simulink model "equation_circle"  (R2021a)
settings: Solver=VariableStepAuto  StartTime=0.0  StopTime=10.0  RelTol=1e-3
libraries: simulink x3
settings Model: Creator=Aula  LastModifiedBy=Aula

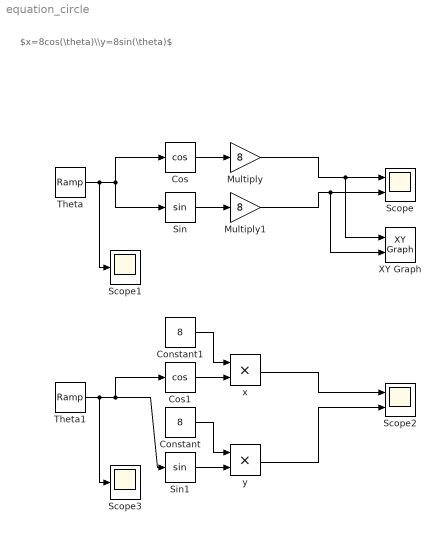
== system equation_circle ==
  note: $x=8cos(\theta)\\y=8sin(\theta)$
  Constant : Constant  Value=8
  Constant1 : Constant  Value=8
  Cos : Trigonometry  Operator=cos
  Cos1 : Trigonometry  Operator=cos
  Multiply : Gain  Gain=8
  Multiply1 : Gain  Gain=8
  Scope : Scope  NumInputPorts=2
  Scope1 : Scope
  Scope2 : Scope  NumInputPorts=2
  Scope3 : Scope
  Sin : Trigonometry
  Sin1 : Trigonometry
  Theta : simulink/Sources/Ramp  slope=1  start=0  InitialOutput=0
  Theta1 : simulink/Sources/Ramp  slope=1  start=0  InitialOutput=0
  XY Graph : simulink/Sinks/XY Graph  xmin=-10  xmax=10  ymin=-10  ymax=010  st=-1
  x : Product
  y : Product
  wires:
  Theta/1 -> Scope1/1, Sin/1, Cos/1
  Cos/1 -> Multiply/1
  Sin/1 -> Multiply1/1
  Multiply/1 -> XY Graph/1, Scope/1
  Multiply1/1 -> XY Graph/2, Scope/2
  Sin1/1 -> y/2
  y/1 -> Scope2/2
  Cos1/1 -> x/2
  x/1 -> Scope2/1
  Theta1/1 -> Scope3/1, Sin1/1, Cos1/1
  Constant1/1 -> x/1
  Constant/1 -> y/1
